simulink model "gm_sampleModel1618_1_sub_sub_sub"  (R2023a)
settings: Solver=VariableStepAuto  StartTime=0.0  StopTime=10.0  RelTol=1e-3
libraries: hdlsllib x7, simulink x3
settings Model: Creator=user1  LastModifiedBy=user1
settings OptimizationCC: BlockReduction=off  ConditionallyExecuteInputs=off
settings DebuggingCC: InheritedTsInSrcMsg=none

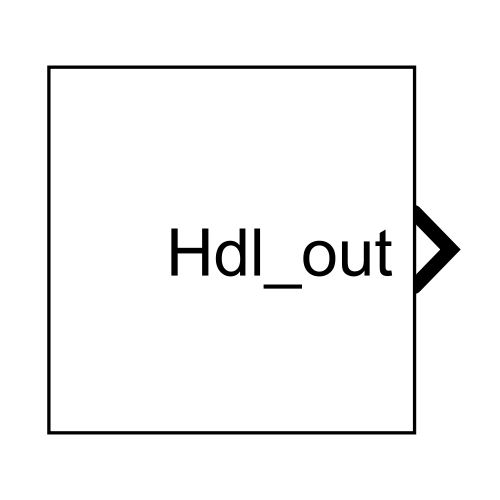
[thumbnail: Simulink's stored preview of the top-level diagram]
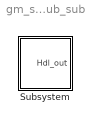
== system gm_sampleModel1618_1_sub_sub_sub ==
  Subsystem : Subsystem

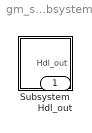
== system gm_sampleModel1618_1_sub_sub_sub/Subsystem ==
  Subsystem : Subsystem
  Hdl_out : Outport  OutDataTypeStr=uint8

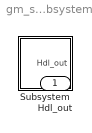
== system gm_sampleModel1618_1_sub_sub_sub/Subsystem/Subsystem ==
  Subsystem : Subsystem
  Hdl_out : Outport  OutDataTypeStr=uint8

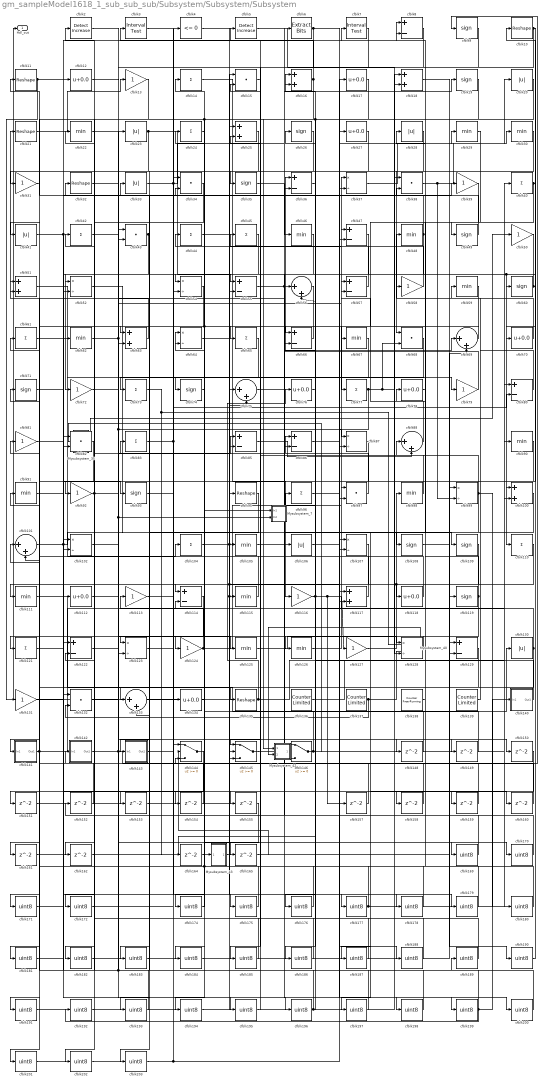
== system gm_sampleModel1618_1_sub_sub_sub/Subsystem/Subsystem/Subsystem ==
  Mysubsystem_35 : Subsystem  TreatAsAtomicUnit=on  RTWFcnName=Mysubsystem_35
      settings: RTWFcnNameOpts=User specified  RTWFileNameOpts=Use function name
  Mysubsystem_40 : Subsystem  TreatAsAtomicUnit=on  RTWFcnName=Mysubsystem_40
      settings: RTWFcnNameOpts=User specified  RTWFileNameOpts=Use function name
  Mysubsystem_42 : Subsystem  TreatAsAtomicUnit=on  RTWFcnName=Mysubsystem_42
      settings: RTWFcnNameOpts=User specified  RTWFileNameOpts=Use function name
  Mysubsystem_43 : Subsystem  TreatAsAtomicUnit=on  RTWFcnName=Mysubsystem_43
      settings: RTWFcnNameOpts=User specified  RTWFileNameOpts=Use function name
  Mysubsystem_7 : Subsystem  TreatAsAtomicUnit=on  RTWFcnName=Mysubsystem_7
      settings: RTWFcnNameOpts=User specified  RTWFileNameOpts=Use function name
  cfblk{10..11,21,32,95,135} (6 alike) : Reshape
  cfblk{16,18,25,51,63,100,117} (7 alike) : Sum  OutDataTypeStr=uint8
  cfblk{56,69,75,88,101,133} (6 alike) : Sum  Inputs=|++  OutDataTypeStr=uint8
  cfblk{37,52,54,64,87,99,102,107,123,128} (10 alike) : Product  Inputs=*/  OutDataTypeStr=uint8  RndMeth=Zero  SaturateOnIntegerOverflow=on
  cfblk{14,24,40,42,44..45,61,65,73,77,83,96,104,110,121} (15 alike) : Sum  Inputs=+  OutDataTypeStr=uint8
  cfblk{22,29..30,46,48,59,62,67,90..91,98,105,111,115,125..126} (16 alike) : MinMax  OutDataTypeStr=uint8
  cfblk{20,23,28,33,41,106,130} (7 alike) : Abs  OutDataTypeStr=uint8  SaturateOnIntegerOverflow=off
  cfblk{9,19,26,35,49,60,71,74,93,108..109,119} (12 alike) : Signum
  cfblk{12,17,27,70,76,78,112,118,134} (9 alike) : Bias  Bias=0.0  SaturateOnIntegerOverflow=off
  cfblk{13,31,39,50,58,72,79,81,92,113,116,124,127,131} (14 alike) : Gain  OutDataTypeStr=uint8
  cfblk{8,36,47,55,57,66,80,85..86,114,122,129} (12 alike) : Sum  Inputs=+-  OutDataTypeStr=uint8
  cfblk{15,34,38,43,68,82,97,132} (8 alike) : DotProduct  OutDataTypeStr=uint8
  cfblk136 : hdlsllib/Sources/Counter Limited  uplimit=7  tsamp=-1
  cfblk137 : hdlsllib/Sources/Counter Limited  uplimit=7  tsamp=-1
  cfblk138 : hdlsllib/Sources/Counter Free-Running  NumBits=16  tsamp=-1
  cfblk139 : hdlsllib/Sources/Counter Limited  uplimit=7  tsamp=-1
  cfblk140 : Subsystem
      settings: LibrarySourceBlock=|
      | hdlsllib/Ports &
      | Subsystems/Subsystem
  cfblk141 : Subsystem
      settings: LibrarySourceBlock=|
      | hdlsllib/Ports &
      | Subsystems/Subsystem
  cfblk142 : Subsystem
      settings: LibrarySourceBlock=|
      | hdlsllib/Ports &
      | Subsystems/Subsystem
  cfblk143 : Subsystem
      settings: LibrarySourceBlock=|
      | hdlsllib/Ports &
      | Subsystems/Subsystem
  cfblk144 : Switch  OutDataTypeStr=uint8  SaturateOnIntegerOverflow=off  InputSameDT=off
  cfblk145 : Switch  OutDataTypeStr=uint8  SaturateOnIntegerOverflow=off  InputSameDT=off
  cfblk146 : Switch  OutDataTypeStr=uint8  SaturateOnIntegerOverflow=off  InputSameDT=off
  cfblk{148..155,157..162,164..165} (16 alike) : Delay  SampleTime=1
  cfblk{169..172,174..203} (34 alike) : DataTypeConversion  OutDataTypeStr=uint8  SaturateOnIntegerOverflow=off  RndMeth=Floor
  cfblk2 : simulink/Logic and Bit Operations/Detect Increase  vinit=0.0  OutDataTypeStr=uint8
      settings: LibrarySourceBlock=|
      | hdlsllib/Logic and Bit
      | Operations/Detect
      | Increase
  cfblk3 : hdlsllib/Logic and Bit Operations/Interval Test  IntervalClosedRight=on  uplimit=0.5  IntervalClosedLeft=on  lowlimit=-0.5  OutDataTypeStr=uint8
  cfblk4 : hdlsllib/Logic and Bit Operations/Compare To Zero  relop=<=  OutDataTypeStr=uint8
  cfblk5 : simulink/Logic and Bit Operations/Detect Increase  vinit=0.0  OutDataTypeStr=uint8
      settings: LibrarySourceBlock=|
      | hdlsllib/Logic and Bit
      | Operations/Detect
      | Increase
  cfblk6 : simulink/Logic and Bit Operations/Extract Bits  bitsToExtract=Upper half  numBits=8  bitIdxRange=[0 7]  outScalingMode=Preserve fixed-point scaling
      settings: LibrarySourceBlock=|
      | hdlsllib/Logic and Bit
      | Operations/Extract Bits
  cfblk7 : hdlsllib/Logic and Bit Operations/Interval Test  IntervalClosedRight=on  uplimit=0.5  IntervalClosedLeft=on  lowlimit=-0.5  OutDataTypeStr=uint8
  Hdl_out : Outport  OutDataTypeStr=uint8
  wires:
  Mysubsystem_43/1(Out1) -> cfblk144/2
  Mysubsystem_42/1(Out1) -> Mysubsystem_35/1(In1)
  Mysubsystem_40/1(Out1) -> Mysubsystem_42/2(In2)
  cfblk19/1 -> Mysubsystem_42/1(In1)
  Mysubsystem_35/1(Out1) -> cfblk50/1
  cfblk203/1 -> cfblk107/2
  cfblk90/1 -> cfblk203/1
  cfblk202/1 -> cfblk107/1
  cfblk46/1 -> cfblk202/1
  cfblk201/1 -> cfblk34/1, cfblk27/1
  cfblk200/1 -> cfblk91/1
  cfblk199/1 -> cfblk192/1, cfblk189/1, cfblk140/1(In1)
  cfblk198/1 -> cfblk122/2
  cfblk197/1 -> cfblk122/1
  cfblk150/1 -> cfblk197/1
  cfblk196/1 -> cfblk33/1, cfblk26/1
  cfblk195/1 -> cfblk25/2
  cfblk162/1 -> cfblk195/1
  cfblk194/1 -> cfblk25/1
  cfblk110/1 -> cfblk194/1
  cfblk193/1 -> cfblk43/1, cfblk142/1(In1)
  cfblk192/1 -> cfblk18/2
  cfblk191/1 -> cfblk18/1
  cfblk190/1 -> cfblk10/1
  cfblk18/1 -> cfblk190/1
  cfblk189/1 -> cfblk96/1
  cfblk188/1 -> cfblk117/1
  cfblk96/1 -> cfblk188/1
  cfblk187/1 -> cfblk15/2
  cfblk186/1 -> cfblk15/1
  cfblk76/1 -> cfblk186/1
  cfblk185/1 -> cfblk152/1
  cfblk15/1 -> cfblk185/1
  cfblk184/1 -> cfblk129/2
  cfblk24/1 -> cfblk184/1
  cfblk183/1 -> cfblk129/1
  cfblk153/1 -> cfblk183/1
  cfblk182/1 -> cfblk115/1, cfblk95/1
  cfblk181/1 -> cfblk102/2
  cfblk180/1 -> cfblk102/1
  cfblk179/1 -> cfblk78/1
  cfblk102/1 -> cfblk179/1
  cfblk178/1 -> cfblk81/1
  cfblk177/1 -> cfblk32/1, cfblk40/1
  cfblk176/1 -> cfblk113/1
  cfblk67/1 -> cfblk176/1
  cfblk175/1 -> cfblk132/1, cfblk14/1
  cfblk174/1 -> cfblk144/3
  cfblk155/1 -> cfblk174/1
  cfblk172/1 -> cfblk144/1
  cfblk114/1 -> cfblk172/1
  cfblk171/1 -> cfblk82/2
  cfblk144/1 -> cfblk171/1
  cfblk170/1 -> cfblk42/1
  cfblk108/1 -> cfblk170/1
  cfblk169/1 -> cfblk146/1
  cfblk42/1 -> cfblk169/1
  cfblk165/1 -> cfblk119/1
  cfblk143/1(Out1) -> cfblk165/1
  cfblk164/1 -> cfblk47/2
  cfblk34/1 -> cfblk162/1
  cfblk161/1 -> cfblk69/2
  cfblk54/1 -> cfblk161/1
  cfblk160/1 -> cfblk82/1
  cfblk32/1 -> cfblk160/1
  cfblk159/1 -> cfblk133/2
  cfblk12/1 -> cfblk159/1
  cfblk158/1 -> cfblk64/2
  cfblk132/1 -> cfblk158/1
  cfblk157/1 -> cfblk146/2
  cfblk154/1 -> cfblk101/1
  cfblk68/1 -> cfblk154/1
  cfblk121/1 -> cfblk153/1
  cfblk152/1 -> cfblk51/2
  cfblk151/1 -> cfblk75/1
  cfblk44/1 -> cfblk150/1
  cfblk149/1 -> cfblk114/2
  cfblk112/1 -> cfblk149/1
  cfblk148/1 -> cfblk66/2
  cfblk130/1 -> cfblk86/1, cfblk181/1
  cfblk119/1 -> cfblk143/1(In1), cfblk38/2
  cfblk97/1 -> cfblk22/1
  cfblk35/1 -> cfblk46/1
  cfblk29/1 -> cfblk49/1
  cfblk113/1 -> cfblk175/1
  cfblk58/1 -> cfblk45/1
  cfblk25/1 -> cfblk193/1
  cfblk72/1 -> cfblk23/1
  cfblk95/1 -> cfblk123/1
  cfblk26/1 -> cfblk141/1(In1)
  cfblk81/1 -> cfblk177/1
  cfblk74/1 -> cfblk124/1
  cfblk142/1(Out1) -> cfblk9/1, cfblk85/1
  cfblk137/1 -> Mysubsystem_40/2(In2), cfblk132/2
  cfblk13/1 -> cfblk52/1
  cfblk55/1 -> cfblk19/1, cfblk198/1
  cfblk33/1 -> cfblk6/1, cfblk87/2
  cfblk5/1 -> cfblk128/2
  cfblk6/1 -> cfblk35/1, cfblk200/1
  cfblk82/1 -> cfblk101/2
  cfblk47/1 -> cfblk55/2
  cfblk36/1 -> cfblk16/2
  cfblk104/1 -> cfblk105/1, cfblk178/1
  cfblk64/1 -> cfblk47/1
  cfblk41/1 -> cfblk93/1, cfblk34/2
  cfblk145/1 -> cfblk97/1
  cfblk27/1 -> cfblk114/1
  cfblk85/1 -> cfblk88/2
  cfblk69/1 -> cfblk66/1
  cfblk133/1 -> cfblk39/1
  cfblk87/1 -> cfblk92/1
  cfblk62/1 -> cfblk56/1, cfblk79/1
  cfblk80/1 -> cfblk58/1
  cfblk40/1 -> cfblk67/1, cfblk70/1
  cfblk4/1 -> cfblk145/3, cfblk117/2
  cfblk140/1(Out1) -> cfblk16/1
  cfblk22/1 -> Mysubsystem_7/2(In2), cfblk148/1
  cfblk3/1 -> cfblk145/2
  cfblk117/1 -> cfblk71/1
  cfblk93/1 -> cfblk80/2
  cfblk116/1 -> cfblk127/1, cfblk157/1, cfblk56/2
  cfblk2/1 -> cfblk125/1, cfblk86/2
  cfblk128/1 -> cfblk121/1
  cfblk79/1 -> cfblk36/2
  cfblk16/1 -> cfblk3/1, cfblk135/1
  cfblk8/1 -> cfblk145/1
  cfblk7/1 -> cfblk54/2
  cfblk99/1 -> cfblk5/1, cfblk180/1, cfblk187/1
  cfblk60/1 -> cfblk54/1, cfblk100/1
  cfblk30/1 -> cfblk63/2
  cfblk73/1 -> Mysubsystem_40/1(In1), cfblk164/1
  cfblk38/1 -> cfblk20/1, cfblk99/2
  cfblk109/1 -> cfblk118/1, cfblk123/2
  cfblk21/1 -> cfblk13/1
  cfblk9/1 -> cfblk65/1
  cfblk43/1 -> cfblk73/1, cfblk52/2
  cfblk131/1 -> cfblk62/1
  cfblk49/1 -> cfblk36/1
  cfblk136/1 -> cfblk80/1
  cfblk70/1 -> cfblk48/1
  cfblk75/1 -> cfblk69/1
  cfblk65/1 -> cfblk133/1
  cfblk134/1 -> cfblk24/1
  cfblk105/1 -> cfblk7/1
  cfblk123/1 -> cfblk4/1
  cfblk106/1 -> cfblk30/1
  cfblk100/1 -> cfblk106/1
  cfblk118/1 -> cfblk51/1
  cfblk31/1 -> cfblk111/1
  cfblk107/1 -> cfblk201/1
  cfblk20/1 -> Mysubsystem_7/1(In1), cfblk41/1
  cfblk51/1 -> cfblk75/2
  cfblk83/1 -> cfblk87/1, cfblk155/1
  cfblk39/1 -> cfblk108/1
  cfblk122/1 -> cfblk196/1
  cfblk141/1(Out1) -> cfblk90/1, cfblk191/1
  cfblk139/1 -> cfblk59/1
  cfblk125/1 -> cfblk128/1
  cfblk77/1 -> cfblk38/1, cfblk68/2, cfblk97/2
  cfblk91/1 -> cfblk199/1
  cfblk138/1 -> cfblk8/1
  cfblk66/1 -> cfblk63/1
  cfblk17/1 -> Mysubsystem_43/1(In1), cfblk85/2
  cfblk71/1 -> cfblk112/1
  cfblk37/1 -> cfblk29/1
  cfblk10/1 -> cfblk60/1, cfblk43/2
  cfblk88/1 -> cfblk57/1
  cfblk57/1 -> cfblk44/1
  cfblk48/1 -> cfblk11/1, cfblk126/1
  cfblk92/1 -> cfblk2/1, cfblk57/2
  cfblk52/1 -> cfblk134/1
  cfblk78/1 -> cfblk28/1
  cfblk86/1 -> cfblk17/1
  cfblk23/1 -> cfblk55/1, cfblk31/1
  cfblk146/1 -> cfblk64/1, cfblk100/2
  cfblk45/1 -> cfblk72/1
  cfblk98/1 -> cfblk88/1
  cfblk115/1 -> cfblk61/1
  cfblk124/1 -> cfblk37/2, cfblk83/1
  cfblk56/1 -> cfblk74/1, cfblk151/1
  cfblk101/1 -> cfblk109/1, cfblk8/2
  cfblk50/1 -> cfblk110/1, cfblk146/3
  cfblk11/1 -> cfblk131/1, cfblk12/1
  cfblk59/1 -> cfblk77/1
  cfblk127/1 -> cfblk98/1
  cfblk14/1 -> cfblk116/1
  cfblk61/1 -> cfblk104/1
  cfblk111/1 -> cfblk130/1
  cfblk135/1 -> cfblk76/1, cfblk99/1, Hdl_out/1
  cfblk126/1 -> cfblk37/1
  cfblk28/1 -> cfblk68/1
  cfblk129/1 -> cfblk182/1
  cfblk63/1 -> cfblk21/1

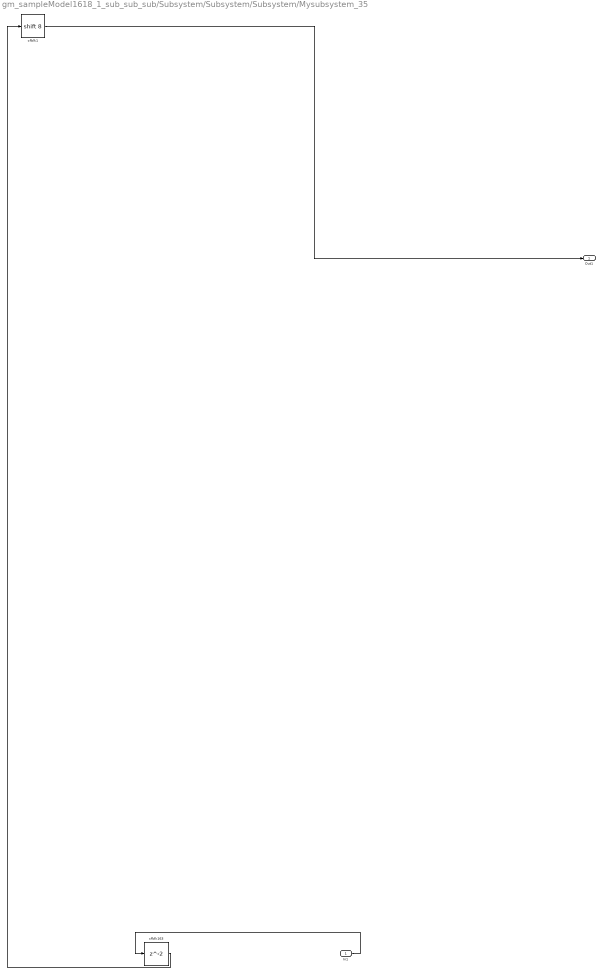
== system gm_sampleModel1618_1_sub_sub_sub/Subsystem/Subsystem/Subsystem/Mysubsystem_35 ==
  In1 : Inport
  cfblk1 : ArithShift  BitShiftNumber=8
  cfblk163 : Delay  SampleTime=1
  Out1 : Outport
  wires:
  cfblk163/1 -> cfblk1/1
  In1/1 -> cfblk163/1
  cfblk1/1 -> Out1/1

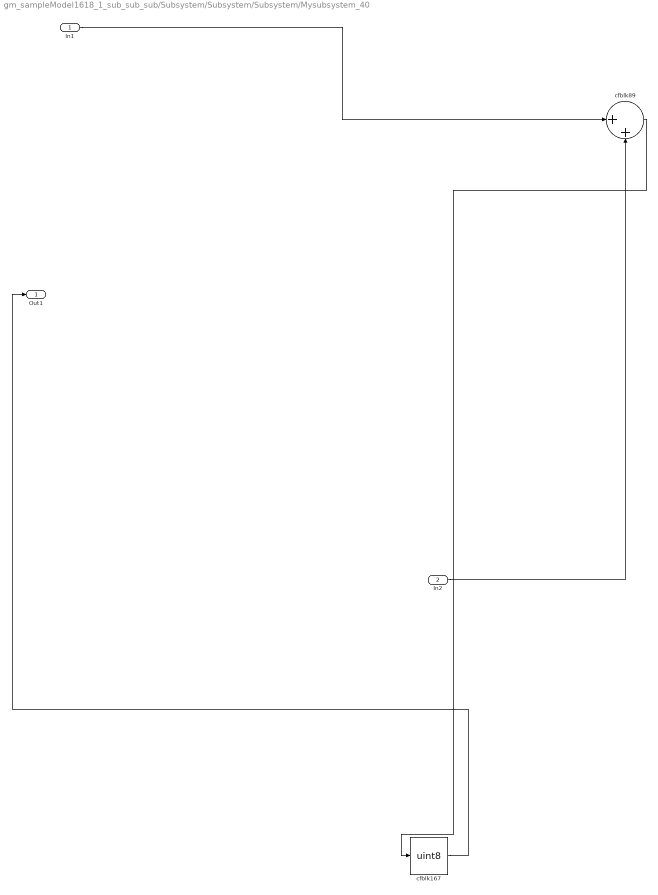
== system gm_sampleModel1618_1_sub_sub_sub/Subsystem/Subsystem/Subsystem/Mysubsystem_40 ==
  In1 : Inport
  In2 : Inport  Port=2
  cfblk167 : DataTypeConversion  OutDataTypeStr=uint8  SaturateOnIntegerOverflow=off  RndMeth=Floor
  cfblk89 : Sum  Inputs=|++
  Out1 : Outport
  wires:
  In2/1 -> cfblk89/2
  cfblk89/1 -> cfblk167/1
  In1/1 -> cfblk89/1
  cfblk167/1 -> Out1/1

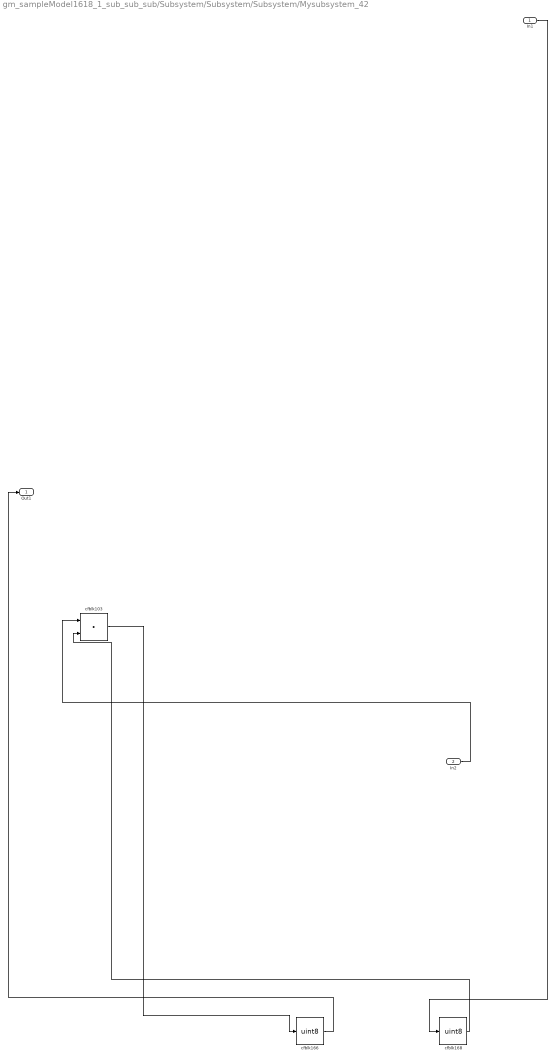
== system gm_sampleModel1618_1_sub_sub_sub/Subsystem/Subsystem/Subsystem/Mysubsystem_42 ==
  In1 : Inport
  In2 : Inport  Port=2
  cfblk103 : DotProduct  OutDataTypeStr=Inherit: Inherit via internal rule
  cfblk166 : DataTypeConversion  OutDataTypeStr=uint8  SaturateOnIntegerOverflow=off  RndMeth=Floor
  cfblk168 : DataTypeConversion  OutDataTypeStr=uint8  SaturateOnIntegerOverflow=off  RndMeth=Floor
  Out1 : Outport
  wires:
  cfblk168/1 -> cfblk103/2
  cfblk166/1 -> Out1/1
  cfblk103/1 -> cfblk166/1
  In1/1 -> cfblk168/1
  In2/1 -> cfblk103/1

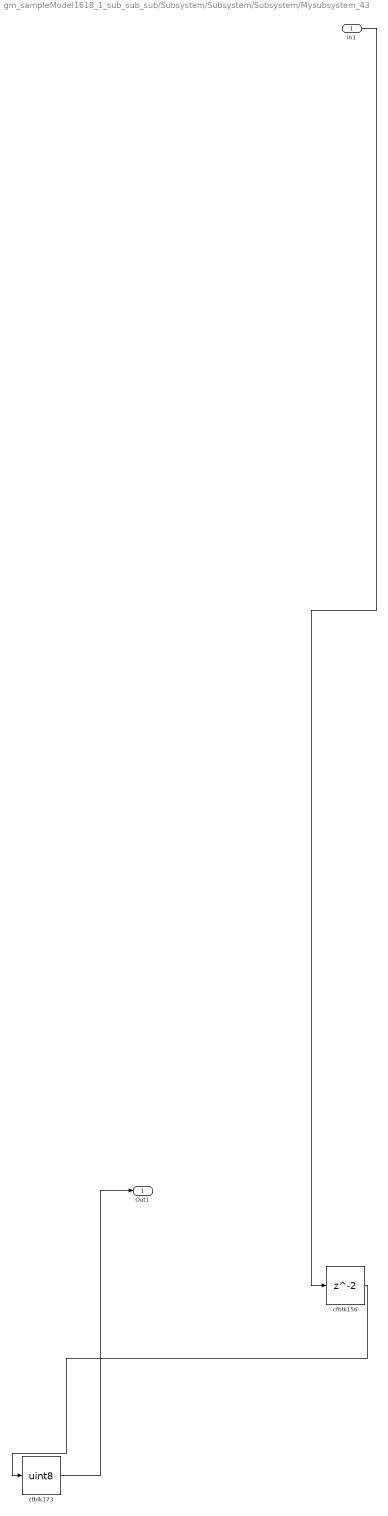
== system gm_sampleModel1618_1_sub_sub_sub/Subsystem/Subsystem/Subsystem/Mysubsystem_43 ==
  In1 : Inport
  cfblk156 : Delay  SampleTime=1
  cfblk173 : DataTypeConversion  OutDataTypeStr=uint8  SaturateOnIntegerOverflow=off  RndMeth=Floor
  Out1 : Outport
  wires:
  cfblk156/1 -> cfblk173/1
  In1/1 -> cfblk156/1
  cfblk173/1 -> Out1/1

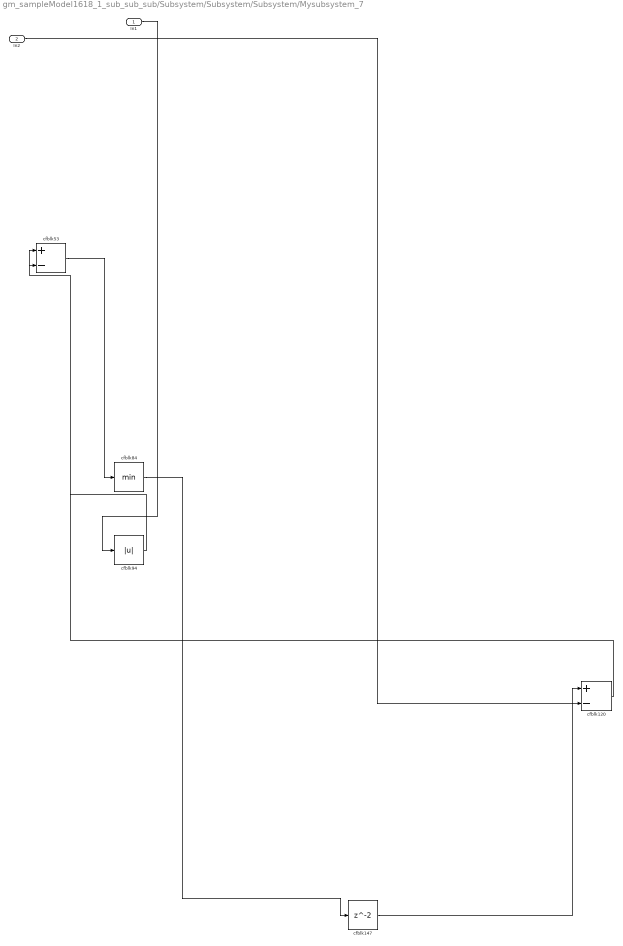
== system gm_sampleModel1618_1_sub_sub_sub/Subsystem/Subsystem/Subsystem/Mysubsystem_7 ==
  In1 : Inport
  In2 : Inport  Port=2
  cfblk120 : Sum  Inputs=+-
  cfblk147 : Delay  SampleTime=1
  cfblk53 : Sum  Inputs=+-
  cfblk84 : MinMax
  cfblk94 : Abs  SaturateOnIntegerOverflow=off
  wires:
  cfblk94/1 -> cfblk53/1
  In1/1 -> cfblk94/1
  cfblk120/1 -> cfblk53/2
  cfblk84/1 -> cfblk147/1
  cfblk53/1 -> cfblk84/1
  In2/1 -> cfblk120/2
  cfblk147/1 -> cfblk120/1

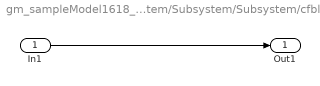
== system gm_sampleModel1618_1_sub_sub_sub/Subsystem/Subsystem/Subsystem/cfblk140 ==
  In1 : Inport
  Out1 : Outport
  wires:
  In1/1 -> Out1/1

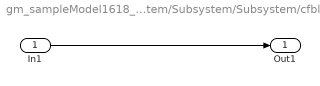
== system gm_sampleModel1618_1_sub_sub_sub/Subsystem/Subsystem/Subsystem/cfblk141 ==
  In1 : Inport
  Out1 : Outport
  wires:
  In1/1 -> Out1/1

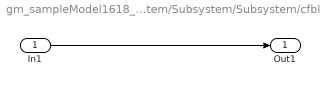
== system gm_sampleModel1618_1_sub_sub_sub/Subsystem/Subsystem/Subsystem/cfblk142 ==
  In1 : Inport
  Out1 : Outport
  wires:
  In1/1 -> Out1/1

== system gm_sampleModel1618_1_sub_sub_sub/Subsystem/Subsystem/Subsystem/cfblk143 ==
  In1 : Inport
  Out1 : Outport
  wires:
  In1/1 -> Out1/1
